simulink model "lag_compensator"  (R2022a)
settings: Solver=VariableStepAuto  StartTime=0.0  StopTime=20  RelTol=1e-3
settings Model: Creator=anthony  LastModifiedBy=anthony

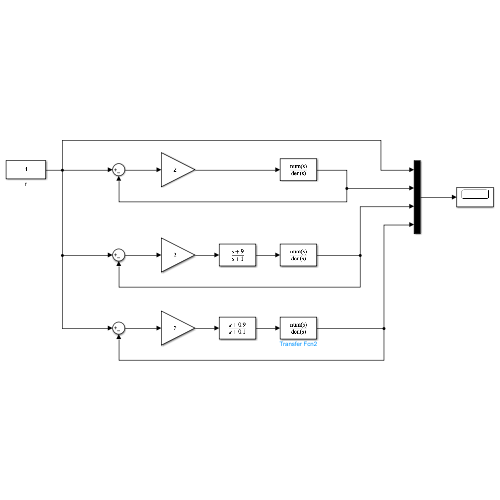
[thumbnail: Simulink's stored preview of the top-level diagram]
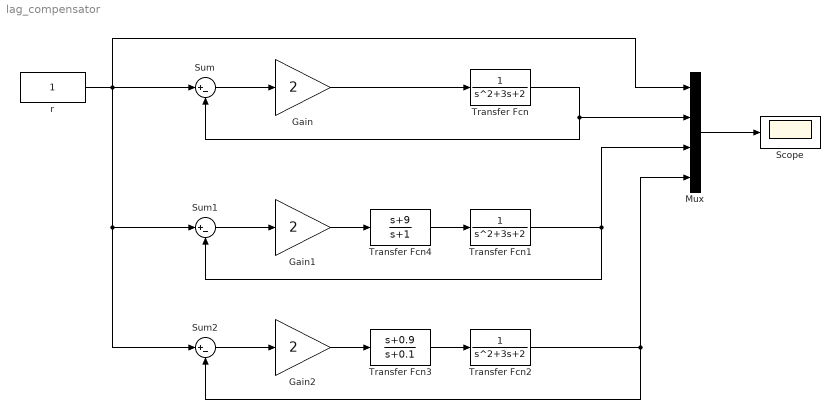
== system lag_compensator ==
  Gain : Gain  Gain=2
  Gain1 : Gain  Gain=2
  Gain2 : Gain  Gain=2
  Mux : Mux
  Scope : Scope
  Sum : Sum  Inputs=|+-
  Sum1 : Sum  Inputs=|+-
  Sum2 : Sum  Inputs=|+-
  Transfer Fcn : TransferFcn  Numerator=[ 1 ]  Denominator=[1 3 2]
  Transfer Fcn1 : TransferFcn  Numerator=[ 1 ]  Denominator=[1 3 2]
  Transfer Fcn2 : TransferFcn  Numerator=[ 1 ]  Denominator=[1 3 2]
  Transfer Fcn3 : TransferFcn  Numerator=[ 1 0.9 ]  Denominator=[1 0.1]
  Transfer Fcn4 : TransferFcn  Numerator=[ 1 9 ]  Denominator=[1 1]
  r : Constant
  wires:
  Mux/1 -> Scope/1
  Sum/1 -> Gain/1
  Gain/1 -> Transfer Fcn/1
  Transfer Fcn/1 -> Sum/2, Mux/2
  Transfer Fcn1/1 -> Sum1/2, Mux/3
  Sum1/1 -> Gain1/1
  Sum2/1 -> Gain2/1
  Transfer Fcn2/1 -> Mux/4, Sum2/2
  r/1 -> Sum2/1, Sum1/1, Mux/1, Sum/1
  Gain2/1 -> Transfer Fcn3/1
  Transfer Fcn3/1 -> Transfer Fcn2/1
  Gain1/1 -> Transfer Fcn4/1
  Transfer Fcn4/1 -> Transfer Fcn1/1
